simulink model "massSpringDamper3"  (R2023a)
settings: Solver=ode4  StartTime=0.0  StopTime=10  FixedStep=0.2  RelTol=1e-3
values from neighbouring files (symbols this model uses):
  b = 0.5    [MSD_variables.m]
  k = 0.5    [MSD_variables.m]
  m = 4    [MSD_variables.m]
settings Model: Creator=kaiad  LastModifiedBy=kaiad
settings DataIOCC: ExternalInput=testSignal2_csv.getElement(1)  LoadExternalInput=on
settings OptimizationCC: ReuseModelBlockBuffer=off

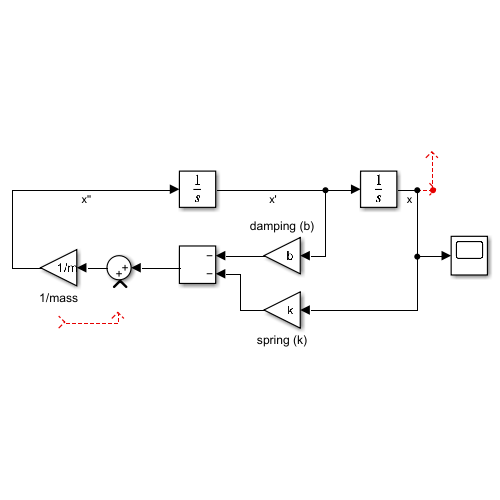
[thumbnail: Simulink's stored preview of the top-level diagram]
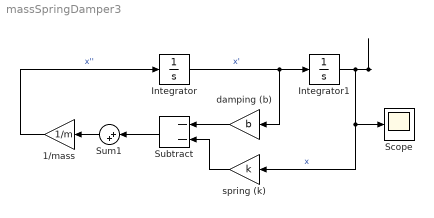
== system massSpringDamper3 ==
  1/mass : Gain  Gain=1/m
  Integrator : Integrator  InitialCondition=2
  Integrator1 : Integrator  InitialCondition=2
  Scope : Scope
  Subtract : Sum  Inputs=--
  Sum1 : Sum  Inputs=|++
  damping (b) : Gain  Gain=b
  spring (k) : Gain  Gain=k
  wires:
  Integrator/1 -> Integrator1/1, damping (b)/1  "x'"
  Integrator1/1 -> Scope/1, spring (k)/1  "x"
  1/mass/1 -> Integrator/1  "x''"
  spring (k)/1 -> Subtract/2
  damping (b)/1 -> Subtract/1
  Subtract/1 -> Sum1/1
  Sum1/1 -> 1/mass/1
  ? -> ?
